simulink model "uwb_re_blackbox"  (Simulink 8.0)
settings: Solver=ode45  StartTime=0.0  StopTime=330  RelTol=1e-3
InitFcn:
  | set_channel;
  | Int_Data_input;
StopFcn:
  | abc=1;
undefined symbols (not defined in the file or in its folder): rsgenpoly
libraries: commutil2 x88, simulink x53, dspmtrx3 x33, dspindex x16, xbsIndex_r4 x12, commcnvcod2 x8, commblkcod2 x8, dspsigops x2, commsink2 x2, commchan3 x1
(part 2 of 5)

== system uwb_re_blackbox/Subsystem2/Creat n_re/delay transmition/hang tram ==
  In1 : Inport
  Integer Delay : Delay  DelayLength=100
  Integer Delay1 : Delay  DelayLength=200
  Integer Delay2 : Delay  DelayLength=300
  Integer Delay3 : Delay  DelayLength=400
  Integer Delay4 : Delay  DelayLength=500
  Integer Delay5 : Delay  DelayLength=600
  Integer Delay6 : Delay  DelayLength=700
  Integer Delay7 : Delay  DelayLength=800
  Integer Delay8 : Delay  DelayLength=900
  Out1 : Outport
  Out2 : Outport  Port=2
  Out3 : Outport  Port=3
  Out4 : Outport  Port=4
  Out5 : Outport  Port=5
  Out6 : Outport  Port=6
  Out7 : Outport  Port=7
  Out8 : Outport  Port=8
  Out9 : Outport  Port=9
  Out10 : Outport  Port=10
  wires:
  In1/1 -> Integer Delay7/1, Integer Delay8/1, Integer Delay6/1, Integer Delay5/1, Integer Delay4/1, Integer Delay3/1, Integer Delay2/1, Integer Delay1/1, Out1/1, Integer Delay/1
  Integer Delay/1 -> Out2/1
  Integer Delay1/1 -> Out3/1
  Integer Delay2/1 -> Out4/1
  Integer Delay3/1 -> Out5/1
  Integer Delay4/1 -> Out6/1
  Integer Delay5/1 -> Out7/1
  Integer Delay6/1 -> Out8/1
  Integer Delay7/1 -> Out9/1
  Integer Delay8/1 -> Out10/1

== system uwb_re_blackbox/Subsystem2/Creat n_re/delay transmition/tach delay ==
  delay : Inport
  Add : Sum  Inputs=+-  SampleTime=3.3/31488
  Add1 : Sum  Inputs=+--
  Add2 : Sum  Inputs=+-  SampleTime=3.3/31488
  Constant1 : Constant  Value=100
  Constant2 : Constant  Value=10
  Constant3 : Constant  Value=1000
  Gain : Gain  Gain=1/100  SampleTime=3.3/31488
  Gain1 : Gain  Gain=1/10  SampleTime=3.3/31488
  Gain2 : Gain  Gain=1/1000  SampleTime=3.3/31488
  Product : Product  SampleTime=3.3/31488  RndMeth=Zero
  Product1 : Product  SampleTime=3.3/31488  RndMeth=Zero
  Product2 : Product  SampleTime=3.3/31488  RndMeth=Zero
  Rounding Function : Rounding
  Rounding Function1 : Rounding  SampleTime=3.3/31488
  Rounding Function2 : Rounding  SampleTime=3.3/31488
  donvi : Outport
  chuc : Outport  Port=2
  Tram : Outport  Port=3
  Nghin : Outport  Port=4
  tre kenh : Outport  Port=5
  wires:
  Product1/1 -> Add1/3
  Constant2/1 -> Product1/2
  Rounding Function1/1 -> Product1/1, chuc/1
  Gain1/1 -> Rounding Function1/1
  Add/1 -> Gain1/1
  Product/1 -> Add/2, Add1/2
  Constant1/1 -> Product/2
  Rounding Function/1 -> Product/1, Tram/1
  Gain/1 -> Rounding Function/1
  Add2/1 -> Gain/1, Add/1, Add1/1
  Gain2/1 -> Rounding Function2/1
  Rounding Function2/1 -> Product2/1, Nghin/1
  delay/1 -> Add2/1, Gain2/1, tre kenh/1
  Constant3/1 -> Product2/2
  Product2/1 -> Add2/2
  Add1/1 -> donvi/1

== system uwb_re_blackbox/Subsystem2/Transmit2/PHR _PSDU/General PHR1 ==
  note: CREAT BLOCK PHR
      | R1 = 0, R0 = 1, P1 = 0, P0 = 0
      | Noctet = N/8 = 100
  EXIT : Constant  Value=0  VectorParams1D=off  OutDataTypeStr=int8  SampleTime=1  FramePeriod=3.3
      settings: SamplingMode=Frame based
  Matrix Concatenate : Concatenate  NumInputs=19  Mode=Multidimensional array  ConcatenateDimension=2
  Noctet : Constant  Value=42  VectorParams1D=off  OutDataTypeStr=int32  SampleTime=1  FramePeriod=3.3
      settings: SamplingMode=Frame based
  P0 : Constant  Value=0  VectorParams1D=off  OutDataTypeStr=int8  SampleTime=1  FramePeriod=3.3
      settings: SamplingMode=Frame based
  P1 : Constant  Value=0  VectorParams1D=off  OutDataTypeStr=int8  SampleTime=1  FramePeriod=3.3
      settings: SamplingMode=Frame based
  PHR(14-->19)1 : Subsystem
  R0 : Constant  VectorParams1D=off  OutDataTypeStr=int8  SampleTime=1  FramePeriod=3.3
      settings: SamplingMode=Frame based
  R1 : Constant  Value=0  VectorParams1D=off  OutDataTypeStr=int8  SampleTime=1  FramePeriod=3.3
      settings: SamplingMode=Frame based
  RNG : Constant  Value=0  VectorParams1D=off  OutDataTypeStr=int8  SampleTime=1  FramePeriod=3.3
      settings: SamplingMode=Frame based
  de2bi : Subsystem
  select element : dspindex/Multiport Selector  rowsOrCols=Columns  idxCellArray={ 1,2,3,4,5,6,7}  idxErrMode=Clip Index
  PHR : Outport
  wires:
  PHR(14-->19)1/6(C0) -> Matrix Concatenate/19
  PHR(14-->19)1/5(C1) -> Matrix Concatenate/18
  PHR(14-->19)1/4(C2) -> Matrix Concatenate/17
  PHR(14-->19)1/3(C3) -> Matrix Concatenate/16
  PHR(14-->19)1/2(C4) -> Matrix Concatenate/15
  PHR(14-->19)1/1(C5) -> Matrix Concatenate/14
  P0/1 -> PHR(14-->19)1/6(P0), Matrix Concatenate/13
  P1/1 -> PHR(14-->19)1/5(P1), Matrix Concatenate/12
  EXIT/1 -> PHR(14-->19)1/4(EXT), Matrix Concatenate/11
  RNG/1 -> PHR(14-->19)1/3(RNG), Matrix Concatenate/10
  select element/7 -> Matrix Concatenate/9
  select element/6 -> Matrix Concatenate/8
  select element/5 -> Matrix Concatenate/7
  select element/4 -> Matrix Concatenate/6
  select element/3 -> Matrix Concatenate/5
  select element/2 -> Matrix Concatenate/4
  select element/1 -> Matrix Concatenate/3
  R0/1 -> PHR(14-->19)1/1(R0), Matrix Concatenate/2
  R1/1 -> Matrix Concatenate/1, PHR(14-->19)1/2(R1)
  de2bi/1(7bit_PHR) -> PHR(14-->19)1/7(7bit_PHR), select element/1
  Matrix Concatenate/1 -> PHR/1
  Noctet/1 -> de2bi/1(Noctet)

== system uwb_re_blackbox/Subsystem2/Transmit2/PHR _PSDU/Subsystem6 ==
  note: cat 6bit chyen sang he 10,55pt he 10 dc dua qua bo RS Encoder.
      | 9pt cuoi dau ra cua RS Encoder dc chuyen sang bit dau ra
  In1 : Inport
  BIN([55:1:63]) to DEC : commutil2/Integer to Bit Converter  nbits=6  signedInputValues=Unsigned  bitOrder=MSB first  outDtype=int8
  Bi2De : commutil2/Bit to Integer Converter  nbits=6  bitOrder=MSB first  signedOutputValues=Unsigned  outDtype=int8  outDtypeSigned=Inherit via internal rule
  Buffer 48bit : Buffer  N=48
  Buffer 55Dec : Buffer  N=55
  Buffer 6bit : Buffer  N=6
  RS Encoder : commblkcod2/Integer-Input RS Encoder  n=63  k=55  specPrimPoly=off  prPoly=[1 0 1 1]  specGenPoly=off  genPoly=rsgenpoly(7,3)  specPuncture=off  punctVec=[ones(2,1); zeros(2,1)]
  Select [55:1:63] : Selector  NumberOfDimensions=2  InputPortWidth=3  IndexOptions=Index vector (dialog),Index vector (dialog)  Indices=[56 57 58 59 60 61 62 63],1  OutputSizes=1,1
  Out1 : Outport
  wires:
  Buffer 48bit/1 -> Out1/1
  BIN([55:1:63]) to DEC/1 -> Buffer 48bit/1
  Select [55:1:63]/1 -> BIN([55:1:63]) to DEC/1
  RS Encoder/1 -> Select [55:1:63]/1
  In1/1 -> Buffer 6bit/1
  Buffer 55Dec/1 -> RS Encoder/1
  Bi2De/1 -> Buffer 55Dec/1
  Buffer 6bit/1 -> Bi2De/1

== system uwb_re_blackbox/Subsystem2/Transmit2/PHR _PSDU1/General PHR1 ==
  note: CREAT BLOCK PHR
      | R1 = 0, R0 = 1, P1 = 0, P0 = 0
      | Noctet = N/8 = 100
  EXIT : Constant  Value=0  VectorParams1D=off  OutDataTypeStr=int8  SampleTime=1  FramePeriod=3.3
      settings: SamplingMode=Frame based
  Matrix Concatenate : Concatenate  NumInputs=19  Mode=Multidimensional array  ConcatenateDimension=2
  Noctet : Constant  Value=42  VectorParams1D=off  OutDataTypeStr=int32  SampleTime=1  FramePeriod=3.3
      settings: SamplingMode=Frame based
  P0 : Constant  Value=0  VectorParams1D=off  OutDataTypeStr=int8  SampleTime=1  FramePeriod=3.3
      settings: SamplingMode=Frame based
  P1 : Constant  Value=0  VectorParams1D=off  OutDataTypeStr=int8  SampleTime=1  FramePeriod=3.3
      settings: SamplingMode=Frame based
  PHR(14-->19)1 : Subsystem
  R0 : Constant  VectorParams1D=off  OutDataTypeStr=int8  SampleTime=1  FramePeriod=3.3
      settings: SamplingMode=Frame based
  R1 : Constant  Value=0  VectorParams1D=off  OutDataTypeStr=int8  SampleTime=1  FramePeriod=3.3
      settings: SamplingMode=Frame based
  RNG : Constant  Value=0  VectorParams1D=off  OutDataTypeStr=int8  SampleTime=1  FramePeriod=3.3
      settings: SamplingMode=Frame based
  de2bi : Subsystem
  select element : dspindex/Multiport Selector  rowsOrCols=Columns  idxCellArray={ 1,2,3,4,5,6,7}  idxErrMode=Clip Index
  PHR : Outport
  wires:
  Noctet/1 -> de2bi/1(Noctet)
  Matrix Concatenate/1 -> PHR/1
  de2bi/1(7bit_PHR) -> select element/1, PHR(14-->19)1/7(7bit_PHR)
  R1/1 -> Matrix Concatenate/1, PHR(14-->19)1/2(R1)
  R0/1 -> Matrix Concatenate/2, PHR(14-->19)1/1(R0)
  select element/1 -> Matrix Concatenate/3
  select element/2 -> Matrix Concatenate/4
  select element/3 -> Matrix Concatenate/5
  select element/4 -> Matrix Concatenate/6
  select element/5 -> Matrix Concatenate/7
  select element/6 -> Matrix Concatenate/8
  select element/7 -> Matrix Concatenate/9
  RNG/1 -> Matrix Concatenate/10, PHR(14-->19)1/3(RNG)
  EXIT/1 -> Matrix Concatenate/11, PHR(14-->19)1/4(EXT)
  P1/1 -> Matrix Concatenate/12, PHR(14-->19)1/5(P1)
  P0/1 -> Matrix Concatenate/13, PHR(14-->19)1/6(P0)
  PHR(14-->19)1/1(C5) -> Matrix Concatenate/14
  PHR(14-->19)1/2(C4) -> Matrix Concatenate/15
  PHR(14-->19)1/3(C3) -> Matrix Concatenate/16
  PHR(14-->19)1/4(C2) -> Matrix Concatenate/17
  PHR(14-->19)1/5(C1) -> Matrix Concatenate/18
  PHR(14-->19)1/6(C0) -> Matrix Concatenate/19

== system uwb_re_blackbox/Subsystem2/Transmit2/PHR _PSDU1/Subsystem6 ==
  note: cat 6bit chyen sang he 10,55pt he 10 dc dua qua bo RS Encoder.
      | 9pt cuoi dau ra cua RS Encoder dc chuyen sang bit dau ra
  In1 : Inport
  BIN([55:1:63]) to DEC : commutil2/Integer to Bit Converter  nbits=6  signedInputValues=Unsigned  bitOrder=MSB first  outDtype=int8
  Bi2De : commutil2/Bit to Integer Converter  nbits=6  bitOrder=MSB first  signedOutputValues=Unsigned  outDtype=int8  outDtypeSigned=Inherit via internal rule
  Buffer 48bit : Buffer  N=48
  Buffer 55Dec : Buffer  N=55
  Buffer 6bit : Buffer  N=6
  RS Encoder : commblkcod2/Integer-Input RS Encoder  n=63  k=55  specPrimPoly=off  prPoly=[1 0 1 1]  specGenPoly=off  genPoly=rsgenpoly(7,3)  specPuncture=off  punctVec=[ones(2,1); zeros(2,1)]
  Select [55:1:63] : Selector  NumberOfDimensions=2  InputPortWidth=3  IndexOptions=Index vector (dialog),Index vector (dialog)  Indices=[56 57 58 59 60 61 62 63],1  OutputSizes=1,1
  Out1 : Outport
  wires:
  Buffer 6bit/1 -> Bi2De/1
  Bi2De/1 -> Buffer 55Dec/1
  Buffer 55Dec/1 -> RS Encoder/1
  In1/1 -> Buffer 6bit/1
  RS Encoder/1 -> Select [55:1:63]/1
  Select [55:1:63]/1 -> BIN([55:1:63]) to DEC/1
  BIN([55:1:63]) to DEC/1 -> Buffer 48bit/1
  Buffer 48bit/1 -> Out1/1

== system uwb_re_blackbox/Subsystem2/Transmit2/PHR _PSDU2/General PHR1 ==
  note: CREAT BLOCK PHR
      | R1 = 0, R0 = 1, P1 = 0, P0 = 0
      | Noctet = N/8 = 100
  EXIT : Constant  Value=0  VectorParams1D=off  OutDataTypeStr=int8  SampleTime=1  FramePeriod=3.3
      settings: SamplingMode=Frame based
  Matrix Concatenate : Concatenate  NumInputs=19  Mode=Multidimensional array  ConcatenateDimension=2
  Noctet : Constant  Value=42  VectorParams1D=off  OutDataTypeStr=int32  SampleTime=1  FramePeriod=3.3
      settings: SamplingMode=Frame based
  P0 : Constant  Value=0  VectorParams1D=off  OutDataTypeStr=int8  SampleTime=1  FramePeriod=3.3
      settings: SamplingMode=Frame based
  P1 : Constant  Value=0  VectorParams1D=off  OutDataTypeStr=int8  SampleTime=1  FramePeriod=3.3
      settings: SamplingMode=Frame based
  PHR(14-->19)1 : Subsystem
  R0 : Constant  VectorParams1D=off  OutDataTypeStr=int8  SampleTime=1  FramePeriod=3.3
      settings: SamplingMode=Frame based
  R1 : Constant  Value=0  VectorParams1D=off  OutDataTypeStr=int8  SampleTime=1  FramePeriod=3.3
      settings: SamplingMode=Frame based
  RNG : Constant  Value=0  VectorParams1D=off  OutDataTypeStr=int8  SampleTime=1  FramePeriod=3.3
      settings: SamplingMode=Frame based
  de2bi : Subsystem
  select element : dspindex/Multiport Selector  rowsOrCols=Columns  idxCellArray={ 1,2,3,4,5,6,7}  idxErrMode=Clip Index
  PHR : Outport
  wires:
  PHR(14-->19)1/6(C0) -> Matrix Concatenate/19
  PHR(14-->19)1/5(C1) -> Matrix Concatenate/18
  PHR(14-->19)1/4(C2) -> Matrix Concatenate/17
  PHR(14-->19)1/3(C3) -> Matrix Concatenate/16
  PHR(14-->19)1/2(C4) -> Matrix Concatenate/15
  PHR(14-->19)1/1(C5) -> Matrix Concatenate/14
  P0/1 -> PHR(14-->19)1/6(P0), Matrix Concatenate/13
  P1/1 -> PHR(14-->19)1/5(P1), Matrix Concatenate/12
  EXIT/1 -> PHR(14-->19)1/4(EXT), Matrix Concatenate/11
  RNG/1 -> PHR(14-->19)1/3(RNG), Matrix Concatenate/10
  select element/7 -> Matrix Concatenate/9
  select element/6 -> Matrix Concatenate/8
  select element/5 -> Matrix Concatenate/7
  select element/4 -> Matrix Concatenate/6
  select element/3 -> Matrix Concatenate/5
  select element/2 -> Matrix Concatenate/4
  select element/1 -> Matrix Concatenate/3
  R0/1 -> PHR(14-->19)1/1(R0), Matrix Concatenate/2
  R1/1 -> PHR(14-->19)1/2(R1), Matrix Concatenate/1
  de2bi/1(7bit_PHR) -> PHR(14-->19)1/7(7bit_PHR), select element/1
  Matrix Concatenate/1 -> PHR/1
  Noctet/1 -> de2bi/1(Noctet)

== system uwb_re_blackbox/Subsystem2/Transmit2/PHR _PSDU2/Subsystem6 ==
  note: cat 6bit chyen sang he 10,55pt he 10 dc dua qua bo RS Encoder.
      | 9pt cuoi dau ra cua RS Encoder dc chuyen sang bit dau ra
  In1 : Inport
  BIN([55:1:63]) to DEC : commutil2/Integer to Bit Converter  nbits=6  signedInputValues=Unsigned  bitOrder=MSB first  outDtype=int8
  Bi2De : commutil2/Bit to Integer Converter  nbits=6  bitOrder=MSB first  signedOutputValues=Unsigned  outDtype=int8  outDtypeSigned=Inherit via internal rule
  Buffer 48bit : Buffer  N=48
  Buffer 55Dec : Buffer  N=55
  Buffer 6bit : Buffer  N=6
  RS Encoder : commblkcod2/Integer-Input RS Encoder  n=63  k=55  specPrimPoly=off  prPoly=[1 0 1 1]  specGenPoly=off  genPoly=rsgenpoly(7,3)  specPuncture=off  punctVec=[ones(2,1); zeros(2,1)]
  Select [55:1:63] : Selector  NumberOfDimensions=2  InputPortWidth=3  IndexOptions=Index vector (dialog),Index vector (dialog)  Indices=[56 57 58 59 60 61 62 63],1  OutputSizes=1,1
  Out1 : Outport
  wires:
  Buffer 48bit/1 -> Out1/1
  BIN([55:1:63]) to DEC/1 -> Buffer 48bit/1
  Select [55:1:63]/1 -> BIN([55:1:63]) to DEC/1
  RS Encoder/1 -> Select [55:1:63]/1
  In1/1 -> Buffer 6bit/1
  Buffer 55Dec/1 -> RS Encoder/1
  Bi2De/1 -> Buffer 55Dec/1
  Buffer 6bit/1 -> Bi2De/1

== system uwb_re_blackbox/Subsystem2/Transmit2/PHR _PSDU3/General PHR1 ==
  note: CREAT BLOCK PHR
      | R1 = 0, R0 = 1, P1 = 0, P0 = 0
      | Noctet = N/8 = 100
  EXIT : Constant  Value=0  VectorParams1D=off  OutDataTypeStr=int8  SampleTime=1  FramePeriod=3.3
      settings: SamplingMode=Frame based
  Matrix Concatenate : Concatenate  NumInputs=19  Mode=Multidimensional array  ConcatenateDimension=2
  Noctet : Constant  Value=42  VectorParams1D=off  OutDataTypeStr=int32  SampleTime=1  FramePeriod=3.3
      settings: SamplingMode=Frame based
  P0 : Constant  Value=0  VectorParams1D=off  OutDataTypeStr=int8  SampleTime=1  FramePeriod=3.3
      settings: SamplingMode=Frame based
  P1 : Constant  Value=0  VectorParams1D=off  OutDataTypeStr=int8  SampleTime=1  FramePeriod=3.3
      settings: SamplingMode=Frame based
  PHR(14-->19)1 : Subsystem
  R0 : Constant  VectorParams1D=off  OutDataTypeStr=int8  SampleTime=1  FramePeriod=3.3
      settings: SamplingMode=Frame based
  R1 : Constant  Value=0  VectorParams1D=off  OutDataTypeStr=int8  SampleTime=1  FramePeriod=3.3
      settings: SamplingMode=Frame based
  RNG : Constant  Value=0  VectorParams1D=off  OutDataTypeStr=int8  SampleTime=1  FramePeriod=3.3
      settings: SamplingMode=Frame based
  de2bi : Subsystem
  select element : dspindex/Multiport Selector  rowsOrCols=Columns  idxCellArray={ 1,2,3,4,5,6,7}  idxErrMode=Clip Index
  PHR : Outport
  wires:
  Noctet/1 -> de2bi/1(Noctet)
  Matrix Concatenate/1 -> PHR/1
  de2bi/1(7bit_PHR) -> select element/1, PHR(14-->19)1/7(7bit_PHR)
  R1/1 -> Matrix Concatenate/1, PHR(14-->19)1/2(R1)
  R0/1 -> Matrix Concatenate/2, PHR(14-->19)1/1(R0)
  select element/1 -> Matrix Concatenate/3
  select element/2 -> Matrix Concatenate/4
  select element/3 -> Matrix Concatenate/5
  select element/4 -> Matrix Concatenate/6
  select element/5 -> Matrix Concatenate/7
  select element/6 -> Matrix Concatenate/8
  select element/7 -> Matrix Concatenate/9
  RNG/1 -> Matrix Concatenate/10, PHR(14-->19)1/3(RNG)
  EXIT/1 -> Matrix Concatenate/11, PHR(14-->19)1/4(EXT)
  P1/1 -> Matrix Concatenate/12, PHR(14-->19)1/5(P1)
  P0/1 -> Matrix Concatenate/13, PHR(14-->19)1/6(P0)
  PHR(14-->19)1/1(C5) -> Matrix Concatenate/14
  PHR(14-->19)1/2(C4) -> Matrix Concatenate/15
  PHR(14-->19)1/3(C3) -> Matrix Concatenate/16
  PHR(14-->19)1/4(C2) -> Matrix Concatenate/17
  PHR(14-->19)1/5(C1) -> Matrix Concatenate/18
  PHR(14-->19)1/6(C0) -> Matrix Concatenate/19

== system uwb_re_blackbox/Subsystem2/Transmit2/PHR _PSDU3/Subsystem6 ==
  note: cat 6bit chyen sang he 10,55pt he 10 dc dua qua bo RS Encoder.
      | 9pt cuoi dau ra cua RS Encoder dc chuyen sang bit dau ra
  In1 : Inport
  BIN([55:1:63]) to DEC : commutil2/Integer to Bit Converter  nbits=6  signedInputValues=Unsigned  bitOrder=MSB first  outDtype=int8
  Bi2De : commutil2/Bit to Integer Converter  nbits=6  bitOrder=MSB first  signedOutputValues=Unsigned  outDtype=int8  outDtypeSigned=Inherit via internal rule
  Buffer 48bit : Buffer  N=48
  Buffer 55Dec : Buffer  N=55
  Buffer 6bit : Buffer  N=6
  RS Encoder : commblkcod2/Integer-Input RS Encoder  n=63  k=55  specPrimPoly=off  prPoly=[1 0 1 1]  specGenPoly=off  genPoly=rsgenpoly(7,3)  specPuncture=off  punctVec=[ones(2,1); zeros(2,1)]
  Select [55:1:63] : Selector  NumberOfDimensions=2  InputPortWidth=3  IndexOptions=Index vector (dialog),Index vector (dialog)  Indices=[56 57 58 59 60 61 62 63],1  OutputSizes=1,1
  Out1 : Outport
  wires:
  Buffer 6bit/1 -> Bi2De/1
  Bi2De/1 -> Buffer 55Dec/1
  Buffer 55Dec/1 -> RS Encoder/1
  In1/1 -> Buffer 6bit/1
  RS Encoder/1 -> Select [55:1:63]/1
  Select [55:1:63]/1 -> BIN([55:1:63]) to DEC/1
  BIN([55:1:63]) to DEC/1 -> Buffer 48bit/1
  Buffer 48bit/1 -> Out1/1

== system uwb_re_blackbox/Subsystem2/Transmit2/PHR _PSDU4/General PHR1 ==
  note: CREAT BLOCK PHR
      | R1 = 0, R0 = 1, P1 = 0, P0 = 0
      | Noctet = N/8 = 100
  EXIT : Constant  Value=0  VectorParams1D=off  OutDataTypeStr=int8  SampleTime=1  FramePeriod=3.3
      settings: SamplingMode=Frame based
  Matrix Concatenate : Concatenate  NumInputs=19  Mode=Multidimensional array  ConcatenateDimension=2
  Noctet : Constant  Value=42  VectorParams1D=off  OutDataTypeStr=int32  SampleTime=1  FramePeriod=3.3
      settings: SamplingMode=Frame based
  P0 : Constant  Value=0  VectorParams1D=off  OutDataTypeStr=int8  SampleTime=1  FramePeriod=3.3
      settings: SamplingMode=Frame based
  P1 : Constant  Value=0  VectorParams1D=off  OutDataTypeStr=int8  SampleTime=1  FramePeriod=3.3
      settings: SamplingMode=Frame based
  PHR(14-->19)1 : Subsystem
  R0 : Constant  VectorParams1D=off  OutDataTypeStr=int8  SampleTime=1  FramePeriod=3.3
      settings: SamplingMode=Frame based
  R1 : Constant  Value=0  VectorParams1D=off  OutDataTypeStr=int8  SampleTime=1  FramePeriod=3.3
      settings: SamplingMode=Frame based
  RNG : Constant  Value=0  VectorParams1D=off  OutDataTypeStr=int8  SampleTime=1  FramePeriod=3.3
      settings: SamplingMode=Frame based
  de2bi : Subsystem
  select element : dspindex/Multiport Selector  rowsOrCols=Columns  idxCellArray={ 1,2,3,4,5,6,7}  idxErrMode=Clip Index
  PHR : Outport
  wires:
  Noctet/1 -> de2bi/1(Noctet)
  Matrix Concatenate/1 -> PHR/1
  de2bi/1(7bit_PHR) -> select element/1, PHR(14-->19)1/7(7bit_PHR)
  R1/1 -> Matrix Concatenate/1, PHR(14-->19)1/2(R1)
  R0/1 -> Matrix Concatenate/2, PHR(14-->19)1/1(R0)
  select element/1 -> Matrix Concatenate/3
  select element/2 -> Matrix Concatenate/4
  select element/3 -> Matrix Concatenate/5
  select element/4 -> Matrix Concatenate/6
  select element/5 -> Matrix Concatenate/7
  select element/6 -> Matrix Concatenate/8
  select element/7 -> Matrix Concatenate/9
  RNG/1 -> Matrix Concatenate/10, PHR(14-->19)1/3(RNG)
  EXIT/1 -> Matrix Concatenate/11, PHR(14-->19)1/4(EXT)
  P1/1 -> Matrix Concatenate/12, PHR(14-->19)1/5(P1)
  P0/1 -> Matrix Concatenate/13, PHR(14-->19)1/6(P0)
  PHR(14-->19)1/1(C5) -> Matrix Concatenate/14
  PHR(14-->19)1/2(C4) -> Matrix Concatenate/15
  PHR(14-->19)1/3(C3) -> Matrix Concatenate/16
  PHR(14-->19)1/4(C2) -> Matrix Concatenate/17
  PHR(14-->19)1/5(C1) -> Matrix Concatenate/18
  PHR(14-->19)1/6(C0) -> Matrix Concatenate/19

== system uwb_re_blackbox/Subsystem2/Transmit2/PHR _PSDU4/Subsystem6 ==
  note: cat 6bit chyen sang he 10,55pt he 10 dc dua qua bo RS Encoder.
      | 9pt cuoi dau ra cua RS Encoder dc chuyen sang bit dau ra
  In1 : Inport
  BIN([55:1:63]) to DEC : commutil2/Integer to Bit Converter  nbits=6  signedInputValues=Unsigned  bitOrder=MSB first  outDtype=int8
  Bi2De : commutil2/Bit to Integer Converter  nbits=6  bitOrder=MSB first  signedOutputValues=Unsigned  outDtype=int8  outDtypeSigned=Inherit via internal rule
  Buffer 48bit : Buffer  N=48
  Buffer 55Dec : Buffer  N=55
  Buffer 6bit : Buffer  N=6
  RS Encoder : commblkcod2/Integer-Input RS Encoder  n=63  k=55  specPrimPoly=off  prPoly=[1 0 1 1]  specGenPoly=off  genPoly=rsgenpoly(7,3)  specPuncture=off  punctVec=[ones(2,1); zeros(2,1)]
  Select [55:1:63] : Selector  NumberOfDimensions=2  InputPortWidth=3  IndexOptions=Index vector (dialog),Index vector (dialog)  Indices=[56 57 58 59 60 61 62 63],1  OutputSizes=1,1
  Out1 : Outport
  wires:
  Buffer 6bit/1 -> Bi2De/1
  Bi2De/1 -> Buffer 55Dec/1
  Buffer 55Dec/1 -> RS Encoder/1
  In1/1 -> Buffer 6bit/1
  RS Encoder/1 -> Select [55:1:63]/1
  Select [55:1:63]/1 -> BIN([55:1:63]) to DEC/1
  BIN([55:1:63]) to DEC/1 -> Buffer 48bit/1
  Buffer 48bit/1 -> Out1/1

== system uwb_re_blackbox/Subsystem2/Transmit2/PHR _PSDU5/General PHR1 ==
  note: CREAT BLOCK PHR
      | R1 = 0, R0 = 1, P1 = 0, P0 = 0
      | Noctet = N/8 = 100
  EXIT : Constant  Value=0  VectorParams1D=off  OutDataTypeStr=int8  SampleTime=1  FramePeriod=3.3
      settings: SamplingMode=Frame based
  Matrix Concatenate : Concatenate  NumInputs=19  Mode=Multidimensional array  ConcatenateDimension=2
  Noctet : Constant  Value=42  VectorParams1D=off  OutDataTypeStr=int32  SampleTime=1  FramePeriod=3.3
      settings: SamplingMode=Frame based
  P0 : Constant  Value=0  VectorParams1D=off  OutDataTypeStr=int8  SampleTime=1  FramePeriod=3.3
      settings: SamplingMode=Frame based
  P1 : Constant  Value=0  VectorParams1D=off  OutDataTypeStr=int8  SampleTime=1  FramePeriod=3.3
      settings: SamplingMode=Frame based
  PHR(14-->19)1 : Subsystem
  R0 : Constant  VectorParams1D=off  OutDataTypeStr=int8  SampleTime=1  FramePeriod=3.3
      settings: SamplingMode=Frame based
  R1 : Constant  Value=0  VectorParams1D=off  OutDataTypeStr=int8  SampleTime=1  FramePeriod=3.3
      settings: SamplingMode=Frame based
  RNG : Constant  Value=0  VectorParams1D=off  OutDataTypeStr=int8  SampleTime=1  FramePeriod=3.3
      settings: SamplingMode=Frame based
  de2bi : Subsystem
  select element : dspindex/Multiport Selector  rowsOrCols=Columns  idxCellArray={ 1,2,3,4,5,6,7}  idxErrMode=Clip Index
  PHR : Outport
  wires:
  PHR(14-->19)1/6(C0) -> Matrix Concatenate/19
  PHR(14-->19)1/5(C1) -> Matrix Concatenate/18
  PHR(14-->19)1/4(C2) -> Matrix Concatenate/17
  PHR(14-->19)1/3(C3) -> Matrix Concatenate/16
  PHR(14-->19)1/2(C4) -> Matrix Concatenate/15
  PHR(14-->19)1/1(C5) -> Matrix Concatenate/14
  P0/1 -> PHR(14-->19)1/6(P0), Matrix Concatenate/13
  P1/1 -> PHR(14-->19)1/5(P1), Matrix Concatenate/12
  EXIT/1 -> PHR(14-->19)1/4(EXT), Matrix Concatenate/11
  RNG/1 -> PHR(14-->19)1/3(RNG), Matrix Concatenate/10
  select element/7 -> Matrix Concatenate/9
  select element/6 -> Matrix Concatenate/8
  select element/5 -> Matrix Concatenate/7
  select element/4 -> Matrix Concatenate/6
  select element/3 -> Matrix Concatenate/5
  select element/2 -> Matrix Concatenate/4
  select element/1 -> Matrix Concatenate/3
  R0/1 -> PHR(14-->19)1/1(R0), Matrix Concatenate/2
  R1/1 -> PHR(14-->19)1/2(R1), Matrix Concatenate/1
  de2bi/1(7bit_PHR) -> PHR(14-->19)1/7(7bit_PHR), select element/1
  Matrix Concatenate/1 -> PHR/1
  Noctet/1 -> de2bi/1(Noctet)

== system uwb_re_blackbox/Subsystem2/Transmit2/PHR _PSDU5/Subsystem6 ==
  note: cat 6bit chyen sang he 10,55pt he 10 dc dua qua bo RS Encoder.
      | 9pt cuoi dau ra cua RS Encoder dc chuyen sang bit dau ra
  In1 : Inport
  BIN([55:1:63]) to DEC : commutil2/Integer to Bit Converter  nbits=6  signedInputValues=Unsigned  bitOrder=MSB first  outDtype=int8
  Bi2De : commutil2/Bit to Integer Converter  nbits=6  bitOrder=MSB first  signedOutputValues=Unsigned  outDtype=int8  outDtypeSigned=Inherit via internal rule
  Buffer 48bit : Buffer  N=48
  Buffer 55Dec : Buffer  N=55
  Buffer 6bit : Buffer  N=6
  RS Encoder : commblkcod2/Integer-Input RS Encoder  n=63  k=55  specPrimPoly=off  prPoly=[1 0 1 1]  specGenPoly=off  genPoly=rsgenpoly(7,3)  specPuncture=off  punctVec=[ones(2,1); zeros(2,1)]
  Select [55:1:63] : Selector  NumberOfDimensions=2  InputPortWidth=3  IndexOptions=Index vector (dialog),Index vector (dialog)  Indices=[56 57 58 59 60 61 62 63],1  OutputSizes=1,1
  Out1 : Outport
  wires:
  Buffer 48bit/1 -> Out1/1
  BIN([55:1:63]) to DEC/1 -> Buffer 48bit/1
  Select [55:1:63]/1 -> BIN([55:1:63]) to DEC/1
  RS Encoder/1 -> Select [55:1:63]/1
  In1/1 -> Buffer 6bit/1
  Buffer 55Dec/1 -> RS Encoder/1
  Bi2De/1 -> Buffer 55Dec/1
  Buffer 6bit/1 -> Bi2De/1

== system uwb_re_blackbox/Subsystem2/Transmit2/PHR _PSDU6/General PHR1 ==
  note: CREAT BLOCK PHR
      | R1 = 0, R0 = 1, P1 = 0, P0 = 0
      | Noctet = N/8 = 100
  EXIT : Constant  Value=0  VectorParams1D=off  OutDataTypeStr=int8  SampleTime=1  FramePeriod=3.3
      settings: SamplingMode=Frame based
  Matrix Concatenate : Concatenate  NumInputs=19  Mode=Multidimensional array  ConcatenateDimension=2
  Noctet : Constant  Value=42  VectorParams1D=off  OutDataTypeStr=int32  SampleTime=1  FramePeriod=3.3
      settings: SamplingMode=Frame based
  P0 : Constant  Value=0  VectorParams1D=off  OutDataTypeStr=int8  SampleTime=1  FramePeriod=3.3
      settings: SamplingMode=Frame based
  P1 : Constant  Value=0  VectorParams1D=off  OutDataTypeStr=int8  SampleTime=1  FramePeriod=3.3
      settings: SamplingMode=Frame based
  PHR(14-->19)1 : Subsystem
  R0 : Constant  VectorParams1D=off  OutDataTypeStr=int8  SampleTime=1  FramePeriod=3.3
      settings: SamplingMode=Frame based
  R1 : Constant  Value=0  VectorParams1D=off  OutDataTypeStr=int8  SampleTime=1  FramePeriod=3.3
      settings: SamplingMode=Frame based
  RNG : Constant  Value=0  VectorParams1D=off  OutDataTypeStr=int8  SampleTime=1  FramePeriod=3.3
      settings: SamplingMode=Frame based
  de2bi : Subsystem
  select element : dspindex/Multiport Selector  rowsOrCols=Columns  idxCellArray={ 1,2,3,4,5,6,7}  idxErrMode=Clip Index
  PHR : Outport
  wires:
  Noctet/1 -> de2bi/1(Noctet)
  Matrix Concatenate/1 -> PHR/1
  de2bi/1(7bit_PHR) -> select element/1, PHR(14-->19)1/7(7bit_PHR)
  R1/1 -> Matrix Concatenate/1, PHR(14-->19)1/2(R1)
  R0/1 -> Matrix Concatenate/2, PHR(14-->19)1/1(R0)
  select element/1 -> Matrix Concatenate/3
  select element/2 -> Matrix Concatenate/4
  select element/3 -> Matrix Concatenate/5
  select element/4 -> Matrix Concatenate/6
  select element/5 -> Matrix Concatenate/7
  select element/6 -> Matrix Concatenate/8
  select element/7 -> Matrix Concatenate/9
  RNG/1 -> Matrix Concatenate/10, PHR(14-->19)1/3(RNG)
  EXIT/1 -> Matrix Concatenate/11, PHR(14-->19)1/4(EXT)
  P1/1 -> Matrix Concatenate/12, PHR(14-->19)1/5(P1)
  P0/1 -> Matrix Concatenate/13, PHR(14-->19)1/6(P0)
  PHR(14-->19)1/1(C5) -> Matrix Concatenate/14
  PHR(14-->19)1/2(C4) -> Matrix Concatenate/15
  PHR(14-->19)1/3(C3) -> Matrix Concatenate/16
  PHR(14-->19)1/4(C2) -> Matrix Concatenate/17
  PHR(14-->19)1/5(C1) -> Matrix Concatenate/18
  PHR(14-->19)1/6(C0) -> Matrix Concatenate/19

== system uwb_re_blackbox/Subsystem2/Transmit2/PHR _PSDU6/Subsystem6 ==
  note: cat 6bit chyen sang he 10,55pt he 10 dc dua qua bo RS Encoder.
      | 9pt cuoi dau ra cua RS Encoder dc chuyen sang bit dau ra
  In1 : Inport
  BIN([55:1:63]) to DEC : commutil2/Integer to Bit Converter  nbits=6  signedInputValues=Unsigned  bitOrder=MSB first  outDtype=int8
  Bi2De : commutil2/Bit to Integer Converter  nbits=6  bitOrder=MSB first  signedOutputValues=Unsigned  outDtype=int8  outDtypeSigned=Inherit via internal rule
  Buffer 48bit : Buffer  N=48
  Buffer 55Dec : Buffer  N=55
  Buffer 6bit : Buffer  N=6
  RS Encoder : commblkcod2/Integer-Input RS Encoder  n=63  k=55  specPrimPoly=off  prPoly=[1 0 1 1]  specGenPoly=off  genPoly=rsgenpoly(7,3)  specPuncture=off  punctVec=[ones(2,1); zeros(2,1)]
  Select [55:1:63] : Selector  NumberOfDimensions=2  InputPortWidth=3  IndexOptions=Index vector (dialog),Index vector (dialog)  Indices=[56 57 58 59 60 61 62 63],1  OutputSizes=1,1
  Out1 : Outport
  wires:
  Buffer 6bit/1 -> Bi2De/1
  Bi2De/1 -> Buffer 55Dec/1
  Buffer 55Dec/1 -> RS Encoder/1
  In1/1 -> Buffer 6bit/1
  RS Encoder/1 -> Select [55:1:63]/1
  Select [55:1:63]/1 -> BIN([55:1:63]) to DEC/1
  BIN([55:1:63]) to DEC/1 -> Buffer 48bit/1
  Buffer 48bit/1 -> Out1/1

== system uwb_re_blackbox/Subsystem2/Transmit2/PHR _PSDU7/General PHR1 ==
  note: CREAT BLOCK PHR
      | R1 = 0, R0 = 1, P1 = 0, P0 = 0
      | Noctet = N/8 = 100
  EXIT : Constant  Value=0  VectorParams1D=off  OutDataTypeStr=int8  SampleTime=1  FramePeriod=3.3
      settings: SamplingMode=Frame based
  Matrix Concatenate : Concatenate  NumInputs=19  Mode=Multidimensional array  ConcatenateDimension=2
  Noctet : Constant  Value=42  VectorParams1D=off  OutDataTypeStr=int32  SampleTime=1  FramePeriod=3.3
      settings: SamplingMode=Frame based
  P0 : Constant  Value=0  VectorParams1D=off  OutDataTypeStr=int8  SampleTime=1  FramePeriod=3.3
      settings: SamplingMode=Frame based
  P1 : Constant  Value=0  VectorParams1D=off  OutDataTypeStr=int8  SampleTime=1  FramePeriod=3.3
      settings: SamplingMode=Frame based
  PHR(14-->19)1 : Subsystem
  R0 : Constant  VectorParams1D=off  OutDataTypeStr=int8  SampleTime=1  FramePeriod=3.3
      settings: SamplingMode=Frame based
  R1 : Constant  Value=0  VectorParams1D=off  OutDataTypeStr=int8  SampleTime=1  FramePeriod=3.3
      settings: SamplingMode=Frame based
  RNG : Constant  Value=0  VectorParams1D=off  OutDataTypeStr=int8  SampleTime=1  FramePeriod=3.3
      settings: SamplingMode=Frame based
  de2bi : Subsystem
  select element : dspindex/Multiport Selector  rowsOrCols=Columns  idxCellArray={ 1,2,3,4,5,6,7}  idxErrMode=Clip Index
  PHR : Outport
  wires:
  PHR(14-->19)1/6(C0) -> Matrix Concatenate/19
  PHR(14-->19)1/5(C1) -> Matrix Concatenate/18
  PHR(14-->19)1/4(C2) -> Matrix Concatenate/17
  PHR(14-->19)1/3(C3) -> Matrix Concatenate/16
  PHR(14-->19)1/2(C4) -> Matrix Concatenate/15
  PHR(14-->19)1/1(C5) -> Matrix Concatenate/14
  P0/1 -> PHR(14-->19)1/6(P0), Matrix Concatenate/13
  P1/1 -> PHR(14-->19)1/5(P1), Matrix Concatenate/12
  EXIT/1 -> PHR(14-->19)1/4(EXT), Matrix Concatenate/11
  RNG/1 -> PHR(14-->19)1/3(RNG), Matrix Concatenate/10
  select element/7 -> Matrix Concatenate/9
  select element/6 -> Matrix Concatenate/8
  select element/5 -> Matrix Concatenate/7
  select element/4 -> Matrix Concatenate/6
  select element/3 -> Matrix Concatenate/5
  select element/2 -> Matrix Concatenate/4
  select element/1 -> Matrix Concatenate/3
  R0/1 -> PHR(14-->19)1/1(R0), Matrix Concatenate/2
  R1/1 -> PHR(14-->19)1/2(R1), Matrix Concatenate/1
  de2bi/1(7bit_PHR) -> PHR(14-->19)1/7(7bit_PHR), select element/1
  Matrix Concatenate/1 -> PHR/1
  Noctet/1 -> de2bi/1(Noctet)

== system uwb_re_blackbox/Subsystem2/Transmit2/PHR _PSDU7/Subsystem6 ==
  note: cat 6bit chyen sang he 10,55pt he 10 dc dua qua bo RS Encoder.
      | 9pt cuoi dau ra cua RS Encoder dc chuyen sang bit dau ra
  In1 : Inport
  BIN([55:1:63]) to DEC : commutil2/Integer to Bit Converter  nbits=6  signedInputValues=Unsigned  bitOrder=MSB first  outDtype=int8
  Bi2De : commutil2/Bit to Integer Converter  nbits=6  bitOrder=MSB first  signedOutputValues=Unsigned  outDtype=int8  outDtypeSigned=Inherit via internal rule
  Buffer 48bit : Buffer  N=48
  Buffer 55Dec : Buffer  N=55
  Buffer 6bit : Buffer  N=6
  RS Encoder : commblkcod2/Integer-Input RS Encoder  n=63  k=55  specPrimPoly=off  prPoly=[1 0 1 1]  specGenPoly=off  genPoly=rsgenpoly(7,3)  specPuncture=off  punctVec=[ones(2,1); zeros(2,1)]
  Select [55:1:63] : Selector  NumberOfDimensions=2  InputPortWidth=3  IndexOptions=Index vector (dialog),Index vector (dialog)  Indices=[56 57 58 59 60 61 62 63],1  OutputSizes=1,1
  Out1 : Outport
  wires:
  Buffer 48bit/1 -> Out1/1
  BIN([55:1:63]) to DEC/1 -> Buffer 48bit/1
  Select [55:1:63]/1 -> BIN([55:1:63]) to DEC/1
  RS Encoder/1 -> Select [55:1:63]/1
  In1/1 -> Buffer 6bit/1
  Buffer 55Dec/1 -> RS Encoder/1
  Bi2De/1 -> Buffer 55Dec/1
  Buffer 6bit/1 -> Bi2De/1

== system uwb_re_blackbox/Subsystem2/Transmit2/Spreading/Hop1 ==
  data : Inport
  s : Inport  Port=2
  Gain2 : Gain  Gain=-1  OutDataTypeStr=int8
  Gain4 : Gain  Gain=-1  OutDataTypeStr=int8
  Kron : Subsystem
      mask Display:
      | disp('KRON');
      | 
      | port_label('input',1,'P');
      | port_label('input',2,'-P');
      | port_label('input',3,'sel');
      | port_label('output',1,'burst');
  Kron1 : Subsystem
      mask Display:
      | disp('KRON');
      | 
      | port_label('input',1,'S');
      | port_label('input',2,'-S');
      | port_label('input',3,'sel');
      | port_label('output',1,'signS');
  Subsystem2 : Subsystem
      mask Display: disp('1/2 Frame data pulse')
  Subsystem3 : Subsystem
      mask Display:
      | port_label('input',1,'data_conv');
      | port_label('output',2,'sign');
      | port_label('output',1,'position');
  Subsystem5 : Subsystem
      mask Display:
      | disp('sel position');
      | 
      | port_label('input',1,'position');
      | port_label('input',2,'matrix');
      | port_label('output',1,'mat_po');
  p : Constant  Value=[-0.0022 -0.0103 -0.0386 -0.1133 -0.2542 -0.4160 -0.4388 -0.1363 0.4543 0.9559 0.9559 0.4543 -0.1363 -0.4388 -0.4160 -0.2542 -0.1133 -0.0386 -0.0103 -0.0022]*2^6  VectorParams1D=off  OutDataTypeStr=int8
      mask Display: disp('xung P')
  Hop1 : Outport
  wires:
  data/1 -> Subsystem3/1(In1)
  Subsystem5/1(Out1) -> Hop1/1
  Subsystem3/1(position) -> Subsystem5/1(In1)
  Subsystem2/1(Out1) -> Subsystem5/2(matrix)
  Subsystem3/2(sign) -> Kron1/3(sel)
  s/1 -> Gain2/1, Kron1/1(p)
  Kron/1(burst) -> Subsystem2/1(In1)
  p/1 -> Gain4/1, Kron/1(p)
  Kron1/1(burst) -> Kron/3(sel)
  Gain4/1 -> Kron/2(-p)
  Gain2/1 -> Kron1/2(-p)

== system uwb_re_blackbox/Subsystem2/Transmit2/Spreading/Hop10 ==
  data : Inport
  s : Inport  Port=2
  Gain2 : Gain  Gain=-1  OutDataTypeStr=int8
  Gain4 : Gain  Gain=-1  OutDataTypeStr=int8
  Kron : Subsystem
      mask Display:
      | disp('KRON');
      | 
      | port_label('input',1,'P');
      | port_label('input',2,'-P');
      | port_label('input',3,'sel');
      | port_label('output',1,'burst');
  Kron1 : Subsystem
      mask Display:
      | disp('KRON');
      | 
      | port_label('input',1,'S');
      | port_label('input',2,'-S');
      | port_label('input',3,'sel');
      | port_label('output',1,'signS');
  Subsystem2 : Subsystem
      mask Display: disp('1/2 Frame data pulse')
  Subsystem3 : Subsystem
      mask Display:
      | port_label('input',1,'data_conv');
      | port_label('output',2,'sign');
      | port_label('output',1,'position');
  Subsystem5 : Subsystem
      mask Display:
      | disp('sel position');
      | 
      | port_label('input',1,'position');
      | port_label('input',2,'matrix');
      | port_label('output',1,'mat_po');
  p : Constant  Value=[-0.0022 -0.0103 -0.0386 -0.1133 -0.2542 -0.4160 -0.4388 -0.1363 0.4543 0.9559 0.9559 0.4543 -0.1363 -0.4388 -0.4160 -0.2542 -0.1133 -0.0386 -0.0103 -0.0022]*2^6  VectorParams1D=off  OutDataTypeStr=int8
      mask Display: disp('xung P')
  Hop1 : Outport
  wires:
  Gain2/1 -> Kron1/2(-p)
  Gain4/1 -> Kron/2(-p)
  Kron1/1(burst) -> Kron/3(sel)
  p/1 -> Kron/1(p), Gain4/1
  Kron/1(burst) -> Subsystem2/1(In1)
  s/1 -> Kron1/1(p), Gain2/1
  Subsystem3/2(sign) -> Kron1/3(sel)
  Subsystem2/1(Out1) -> Subsystem5/2(matrix)
  Subsystem3/1(position) -> Subsystem5/1(In1)
  Subsystem5/1(Out1) -> Hop1/1
  data/1 -> Subsystem3/1(In1)

== system uwb_re_blackbox/Subsystem2/Transmit2/Spreading/Hop11 ==
  data : Inport
  s : Inport  Port=2
  Gain2 : Gain  Gain=-1  OutDataTypeStr=int8
  Gain4 : Gain  Gain=-1  OutDataTypeStr=int8
  Kron : Subsystem
      mask Display:
      | disp('KRON');
      | 
      | port_label('input',1,'P');
      | port_label('input',2,'-P');
      | port_label('input',3,'sel');
      | port_label('output',1,'burst');
  Kron1 : Subsystem
      mask Display:
      | disp('KRON');
      | 
      | port_label('input',1,'S');
      | port_label('input',2,'-S');
      | port_label('input',3,'sel');
      | port_label('output',1,'signS');
  Subsystem2 : Subsystem
      mask Display: disp('1/2 Frame data pulse')
  Subsystem3 : Subsystem
      mask Display:
      | port_label('input',1,'data_conv');
      | port_label('output',2,'sign');
      | port_label('output',1,'position');
  Subsystem5 : Subsystem
      mask Display:
      | disp('sel position');
      | 
      | port_label('input',1,'position');
      | port_label('input',2,'matrix');
      | port_label('output',1,'mat_po');
  p : Constant  Value=[-0.0022 -0.0103 -0.0386 -0.1133 -0.2542 -0.4160 -0.4388 -0.1363 0.4543 0.9559 0.9559 0.4543 -0.1363 -0.4388 -0.4160 -0.2542 -0.1133 -0.0386 -0.0103 -0.0022]*2^6  VectorParams1D=off  OutDataTypeStr=int8
      mask Display: disp('xung P')
  Hop1 : Outport
  wires:
  data/1 -> Subsystem3/1(In1)
  Subsystem5/1(Out1) -> Hop1/1
  Subsystem3/1(position) -> Subsystem5/1(In1)
  Subsystem2/1(Out1) -> Subsystem5/2(matrix)
  Subsystem3/2(sign) -> Kron1/3(sel)
  s/1 -> Gain2/1, Kron1/1(p)
  Kron/1(burst) -> Subsystem2/1(In1)
  p/1 -> Gain4/1, Kron/1(p)
  Kron1/1(burst) -> Kron/3(sel)
  Gain4/1 -> Kron/2(-p)
  Gain2/1 -> Kron1/2(-p)

== system uwb_re_blackbox/Subsystem2/Transmit2/Spreading/Hop12 ==
  data : Inport
  s : Inport  Port=2
  Gain2 : Gain  Gain=-1  OutDataTypeStr=int8
  Gain4 : Gain  Gain=-1  OutDataTypeStr=int8
  Kron : Subsystem
      mask Display:
      | disp('KRON');
      | 
      | port_label('input',1,'P');
      | port_label('input',2,'-P');
      | port_label('input',3,'sel');
      | port_label('output',1,'burst');
  Kron1 : Subsystem
      mask Display:
      | disp('KRON');
      | 
      | port_label('input',1,'S');
      | port_label('input',2,'-S');
      | port_label('input',3,'sel');
      | port_label('output',1,'signS');
  Subsystem2 : Subsystem
      mask Display: disp('1/2 Frame data pulse')
  Subsystem3 : Subsystem
      mask Display:
      | port_label('input',1,'data_conv');
      | port_label('output',2,'sign');
      | port_label('output',1,'position');
  Subsystem5 : Subsystem
      mask Display:
      | disp('sel position');
      | 
      | port_label('input',1,'position');
      | port_label('input',2,'matrix');
      | port_label('output',1,'mat_po');
  p : Constant  Value=[-0.0022 -0.0103 -0.0386 -0.1133 -0.2542 -0.4160 -0.4388 -0.1363 0.4543 0.9559 0.9559 0.4543 -0.1363 -0.4388 -0.4160 -0.2542 -0.1133 -0.0386 -0.0103 -0.0022]*2^6  VectorParams1D=off  OutDataTypeStr=int8
      mask Display: disp('xung P')
  Hop1 : Outport
  wires:
  data/1 -> Subsystem3/1(In1)
  Subsystem5/1(Out1) -> Hop1/1
  Subsystem3/1(position) -> Subsystem5/1(In1)
  Subsystem2/1(Out1) -> Subsystem5/2(matrix)
  Subsystem3/2(sign) -> Kron1/3(sel)
  s/1 -> Gain2/1, Kron1/1(p)
  Kron/1(burst) -> Subsystem2/1(In1)
  p/1 -> Gain4/1, Kron/1(p)
  Kron1/1(burst) -> Kron/3(sel)
  Gain4/1 -> Kron/2(-p)
  Gain2/1 -> Kron1/2(-p)

== system uwb_re_blackbox/Subsystem2/Transmit2/Spreading/Hop13 ==
  data : Inport
  s : Inport  Port=2
  Gain2 : Gain  Gain=-1  OutDataTypeStr=int8
  Gain4 : Gain  Gain=-1  OutDataTypeStr=int8
  Kron : Subsystem
      mask Display:
      | disp('KRON');
      | 
      | port_label('input',1,'P');
      | port_label('input',2,'-P');
      | port_label('input',3,'sel');
      | port_label('output',1,'burst');
  Kron1 : Subsystem
      mask Display:
      | disp('KRON');
      | 
      | port_label('input',1,'S');
      | port_label('input',2,'-S');
      | port_label('input',3,'sel');
      | port_label('output',1,'signS');
  Subsystem2 : Subsystem
      mask Display: disp('1/2 Frame data pulse')
  Subsystem3 : Subsystem
      mask Display:
      | port_label('input',1,'data_conv');
      | port_label('output',2,'sign');
      | port_label('output',1,'position');
  Subsystem5 : Subsystem
      mask Display:
      | disp('sel position');
      | 
      | port_label('input',1,'position');
      | port_label('input',2,'matrix');
      | port_label('output',1,'mat_po');
  p : Constant  Value=[-0.0022 -0.0103 -0.0386 -0.1133 -0.2542 -0.4160 -0.4388 -0.1363 0.4543 0.9559 0.9559 0.4543 -0.1363 -0.4388 -0.4160 -0.2542 -0.1133 -0.0386 -0.0103 -0.0022]*2^6  VectorParams1D=off  OutDataTypeStr=int8
      mask Display: disp('xung P')
  Hop1 : Outport
  wires:
  Gain2/1 -> Kron1/2(-p)
  Gain4/1 -> Kron/2(-p)
  Kron1/1(burst) -> Kron/3(sel)
  p/1 -> Kron/1(p), Gain4/1
  Kron/1(burst) -> Subsystem2/1(In1)
  s/1 -> Kron1/1(p), Gain2/1
  Subsystem3/2(sign) -> Kron1/3(sel)
  Subsystem2/1(Out1) -> Subsystem5/2(matrix)
  Subsystem3/1(position) -> Subsystem5/1(In1)
  Subsystem5/1(Out1) -> Hop1/1
  data/1 -> Subsystem3/1(In1)

== system uwb_re_blackbox/Subsystem2/Transmit2/Spreading/Hop14 ==
  data : Inport
  s : Inport  Port=2
  Gain2 : Gain  Gain=-1  OutDataTypeStr=int8
  Gain4 : Gain  Gain=-1  OutDataTypeStr=int8
  Kron : Subsystem
      mask Display:
      | disp('KRON');
      | 
      | port_label('input',1,'P');
      | port_label('input',2,'-P');
      | port_label('input',3,'sel');
      | port_label('output',1,'burst');
  Kron1 : Subsystem
      mask Display:
      | disp('KRON');
      | 
      | port_label('input',1,'S');
      | port_label('input',2,'-S');
      | port_label('input',3,'sel');
      | port_label('output',1,'signS');
  Subsystem2 : Subsystem
      mask Display: disp('1/2 Frame data pulse')
  Subsystem3 : Subsystem
      mask Display:
      | port_label('input',1,'data_conv');
      | port_label('output',2,'sign');
      | port_label('output',1,'position');
  Subsystem5 : Subsystem
      mask Display:
      | disp('sel position');
      | 
      | port_label('input',1,'position');
      | port_label('input',2,'matrix');
      | port_label('output',1,'mat_po');
  p : Constant  Value=[-0.0022 -0.0103 -0.0386 -0.1133 -0.2542 -0.4160 -0.4388 -0.1363 0.4543 0.9559 0.9559 0.4543 -0.1363 -0.4388 -0.4160 -0.2542 -0.1133 -0.0386 -0.0103 -0.0022]*2^6  VectorParams1D=off  OutDataTypeStr=int8
      mask Display: disp('xung P')
  Hop1 : Outport
  wires:
  data/1 -> Subsystem3/1(In1)
  Subsystem5/1(Out1) -> Hop1/1
  Subsystem3/1(position) -> Subsystem5/1(In1)
  Subsystem2/1(Out1) -> Subsystem5/2(matrix)
  Subsystem3/2(sign) -> Kron1/3(sel)
  s/1 -> Gain2/1, Kron1/1(p)
  Kron/1(burst) -> Subsystem2/1(In1)
  p/1 -> Gain4/1, Kron/1(p)
  Kron1/1(burst) -> Kron/3(sel)
  Gain4/1 -> Kron/2(-p)
  Gain2/1 -> Kron1/2(-p)

== system uwb_re_blackbox/Subsystem2/Transmit2/Spreading/Hop15 ==
  data : Inport
  s : Inport  Port=2
  Gain2 : Gain  Gain=-1  OutDataTypeStr=int8
  Gain4 : Gain  Gain=-1  OutDataTypeStr=int8
  Kron : Subsystem
      mask Display:
      | disp('KRON');
      | 
      | port_label('input',1,'P');
      | port_label('input',2,'-P');
      | port_label('input',3,'sel');
      | port_label('output',1,'burst');
  Kron1 : Subsystem
      mask Display:
      | disp('KRON');
      | 
      | port_label('input',1,'S');
      | port_label('input',2,'-S');
      | port_label('input',3,'sel');
      | port_label('output',1,'signS');
  Subsystem2 : Subsystem
      mask Display: disp('1/2 Frame data pulse')
  Subsystem3 : Subsystem
      mask Display:
      | port_label('input',1,'data_conv');
      | port_label('output',2,'sign');
      | port_label('output',1,'position');
  Subsystem5 : Subsystem
      mask Display:
      | disp('sel position');
      | 
      | port_label('input',1,'position');
      | port_label('input',2,'matrix');
      | port_label('output',1,'mat_po');
  p : Constant  Value=[-0.0022 -0.0103 -0.0386 -0.1133 -0.2542 -0.4160 -0.4388 -0.1363 0.4543 0.9559 0.9559 0.4543 -0.1363 -0.4388 -0.4160 -0.2542 -0.1133 -0.0386 -0.0103 -0.0022]*2^6  VectorParams1D=off  OutDataTypeStr=int8
      mask Display: disp('xung P')
  Hop1 : Outport
  wires:
  Gain2/1 -> Kron1/2(-p)
  Gain4/1 -> Kron/2(-p)
  Kron1/1(burst) -> Kron/3(sel)
  p/1 -> Kron/1(p), Gain4/1
  Kron/1(burst) -> Subsystem2/1(In1)
  s/1 -> Kron1/1(p), Gain2/1
  Subsystem3/2(sign) -> Kron1/3(sel)
  Subsystem2/1(Out1) -> Subsystem5/2(matrix)
  Subsystem3/1(position) -> Subsystem5/1(In1)
  Subsystem5/1(Out1) -> Hop1/1
  data/1 -> Subsystem3/1(In1)

== system uwb_re_blackbox/Subsystem2/Transmit2/Spreading/Hop17 ==
  data : Inport
  s : Inport  Port=2
  Gain2 : Gain  Gain=-1  OutDataTypeStr=int8
  Gain4 : Gain  Gain=-1  OutDataTypeStr=int8
  Kron : Subsystem
      mask Display:
      | disp('KRON');
      | 
      | port_label('input',1,'P');
      | port_label('input',2,'-P');
      | port_label('input',3,'sel');
      | port_label('output',1,'burst');
  Kron1 : Subsystem
      mask Display:
      | disp('KRON');
      | 
      | port_label('input',1,'S');
      | port_label('input',2,'-S');
      | port_label('input',3,'sel');
      | port_label('output',1,'signS');
  Subsystem2 : Subsystem
      mask Display: disp('1/2 Frame data pulse')
  Subsystem3 : Subsystem
      mask Display:
      | port_label('input',1,'data_conv');
      | port_label('output',2,'sign');
      | port_label('output',1,'position');
  Subsystem5 : Subsystem
      mask Display:
      | disp('sel position');
      | 
      | port_label('input',1,'position');
      | port_label('input',2,'matrix');
      | port_label('output',1,'mat_po');
  p : Constant  Value=[-0.0022 -0.0103 -0.0386 -0.1133 -0.2542 -0.4160 -0.4388 -0.1363 0.4543 0.9559 0.9559 0.4543 -0.1363 -0.4388 -0.4160 -0.2542 -0.1133 -0.0386 -0.0103 -0.0022]*2^6  VectorParams1D=off  OutDataTypeStr=int8
      mask Display: disp('xung P')
  Hop1 : Outport
  wires:
  Gain2/1 -> Kron1/2(-p)
  Gain4/1 -> Kron/2(-p)
  Kron1/1(burst) -> Kron/3(sel)
  p/1 -> Kron/1(p), Gain4/1
  Kron/1(burst) -> Subsystem2/1(In1)
  s/1 -> Kron1/1(p), Gain2/1
  Subsystem3/2(sign) -> Kron1/3(sel)
  Subsystem2/1(Out1) -> Subsystem5/2(matrix)
  Subsystem3/1(position) -> Subsystem5/1(In1)
  Subsystem5/1(Out1) -> Hop1/1
  data/1 -> Subsystem3/1(In1)

== system uwb_re_blackbox/Subsystem2/Transmit2/Spreading/Hop2 ==
  data : Inport
  s : Inport  Port=2
  Gain2 : Gain  Gain=-1  OutDataTypeStr=int8
  Gain4 : Gain  Gain=-1  OutDataTypeStr=int8
  Kron : Subsystem
      mask Display:
      | disp('KRON');
      | 
      | port_label('input',1,'P');
      | port_label('input',2,'-P');
      | port_label('input',3,'sel');
      | port_label('output',1,'burst');
  Kron1 : Subsystem
      mask Display:
      | disp('KRON');
      | 
      | port_label('input',1,'S');
      | port_label('input',2,'-S');
      | port_label('input',3,'sel');
      | port_label('output',1,'signS');
  Subsystem2 : Subsystem
      mask Display: disp('1/2 Frame data pulse')
  Subsystem3 : Subsystem
      mask Display:
      | port_label('input',1,'data_conv');
      | port_label('output',2,'sign');
      | port_label('output',1,'position');
  Subsystem5 : Subsystem
      mask Display:
      | disp('sel position');
      | 
      | port_label('input',1,'position');
      | port_label('input',2,'matrix');
      | port_label('output',1,'mat_po');
  p : Constant  Value=[-0.0022 -0.0103 -0.0386 -0.1133 -0.2542 -0.4160 -0.4388 -0.1363 0.4543 0.9559 0.9559 0.4543 -0.1363 -0.4388 -0.4160 -0.2542 -0.1133 -0.0386 -0.0103 -0.0022]*2^6  VectorParams1D=off  OutDataTypeStr=int8
      mask Display: disp('xung P')
  Hop1 : Outport
  wires:
  Gain2/1 -> Kron1/2(-p)
  Gain4/1 -> Kron/2(-p)
  Kron1/1(burst) -> Kron/3(sel)
  p/1 -> Kron/1(p), Gain4/1
  Kron/1(burst) -> Subsystem2/1(In1)
  s/1 -> Kron1/1(p), Gain2/1
  Subsystem3/2(sign) -> Kron1/3(sel)
  Subsystem2/1(Out1) -> Subsystem5/2(matrix)
  Subsystem3/1(position) -> Subsystem5/1(In1)
  Subsystem5/1(Out1) -> Hop1/1
  data/1 -> Subsystem3/1(In1)
